simulink model "acionamento_six_step1"  (R2012b)
settings: Solver=ode45  StartTime=0.0  StopTime=1  RelTol=1e-3
libraries: BLDC x3
settings Model: Creator=h3now  LastModifiedBy=h3now

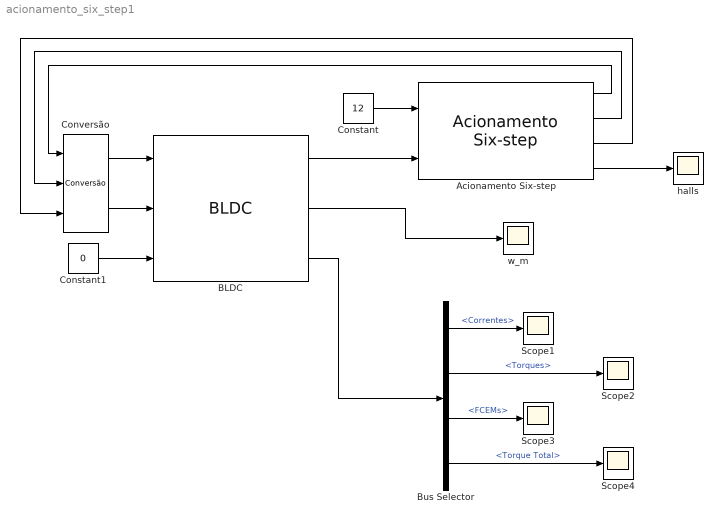
== system acionamento_six_step1 ==
  Acionamento Six-step : BLDC/Acionamento Six-step  P=8
  BLDC : BLDC/BLDC  J=1.39e-6  R=10.1/2  L=2.04/2000  P=8  Kt=15.7e-3/1.19  Ke=15.7e-3/1.19  Kd=0  F_stick=0  F_slip=0  default_fcem=on  fcem_a=fcem_a  fcem_b=fcem_b  fcem_c=fcem_c
  Bus Selector : BusSelector  OutputSignals=Correntes,Torques,FCEMs,Torque Total
  Constant : Constant  Value=12
  Constant1 : Constant  Value=0
  Conversão : BLDC/Conversão
  Scope{1..4} (4 alike) : Scope
      Scope2 settings: SaveName=ScopeData2
      Scope3 settings: SaveName=ScopeData3
      Scope4 settings: SaveName=ScopeData4
  halls : Scope
      settings: SaveName=ScopeData5
  w_m : Scope
  wires:
  BLDC/1 -> Acionamento Six-step/2
  Constant/1 -> Acionamento Six-step/1
  Constant1/1 -> BLDC/3
  BLDC/3 -> Bus Selector/1
  BLDC/2 -> w_m/1
  Bus Selector/1 -> Scope1/1  "<Correntes>"
  Bus Selector/2 -> Scope2/1  "<Torques>"
  Bus Selector/3 -> Scope3/1  "<FCEMs>"
  Bus Selector/4 -> Scope4/1  "<Torque Total>"
  Acionamento Six-step/4 -> halls/1
  Conversão/1 -> BLDC/1
  Conversão/2 -> BLDC/2
  Acionamento Six-step/1 -> Conversão/1
  Acionamento Six-step/2 -> Conversão/2
  Acionamento Six-step/3 -> Conversão/3
